simulink library "modularPlant_cl"  (R2018b)
settings: Solver=VariableStepAuto  StartTime=0.0  StopTime=10.0  RelTol=1e-3
libraries: groundStation_cl x1, tethers_cl x1, vehicle_cl x1, winch_cl x1
settings Model: Creator=mcobb  LastModifiedBy=mcobb

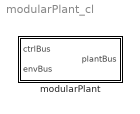
== system modularPlant_cl ==
  modularPlant : Subsystem  VariantControl=VSS_plant_modularPlant

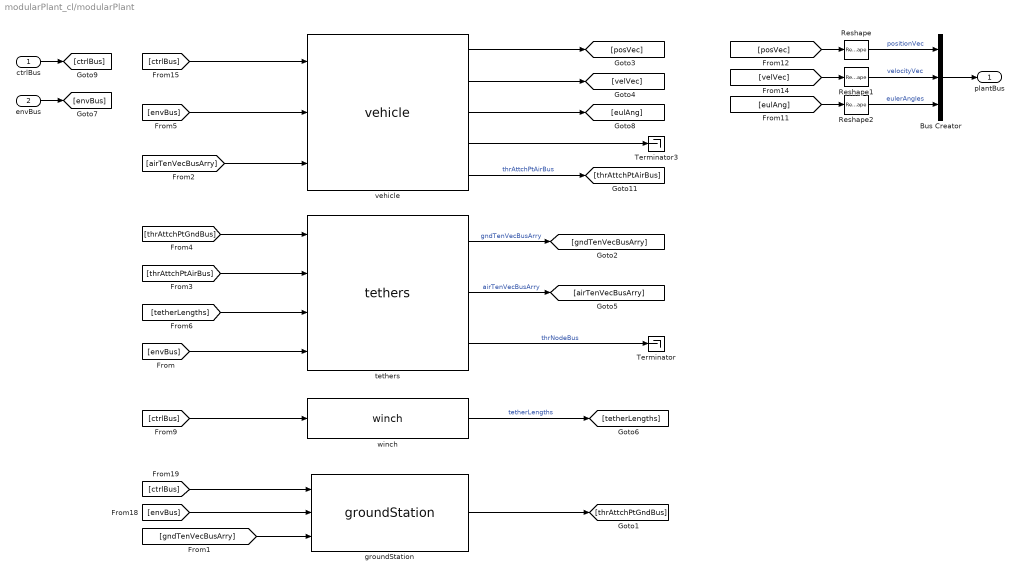
== system modularPlant_cl/modularPlant ==
  ctrlBus : Inport  OutDataTypeStr=Bus: ctrlBus
  envBus : Inport  Port=2  OutDataTypeStr=Bus: envBus
  Bus Creator : BusCreator  Inputs=3  OutDataTypeStr=Bus: plantBus
  Reshape : Reshape  OutputDimensionality=Column vector (2-D)
  Reshape1 : Reshape  OutputDimensionality=Column vector (2-D)
  Reshape2 : Reshape  OutputDimensionality=Column vector (2-D)
  Terminator : Terminator
  Terminator3 : Terminator
  groundStation : groundStation_cl/groundStation  SystemSampleTime=-1
  "tethers " : tethers_cl/tethers  SystemSampleTime=-1
  vehicle : vehicle_cl/vehicle  SystemSampleTime=-1
  winch : winch_cl/winch  SystemSampleTime=-1
  plantBus : Outport  OutDataTypeStr=Bus: plantBus
  wires:
  envBus/1 -> [envBus]
  ctrlBus/1 -> [ctrlBus]
  Bus Creator/1 -> plantBus/1
  Reshape/1 -> Bus Creator/1  "positionVec"
  Reshape2/1 -> Bus Creator/3  "eulerAngles"
  Reshape1/1 -> Bus Creator/2  "velocityVec"
  winch/1 -> [tetherLengths]  "tetherLengths"
  [posVec] -> Reshape/1
  [velVec] -> Reshape1/1
  [eulAng] -> Reshape2/1
  vehicle/3 -> [eulAng]
  vehicle/1 -> [posVec]
  vehicle/5 -> [thrAttchPtAirBus]  "thrAttchPtAirBus"
  vehicle/2 -> [velVec]
  vehicle/4 -> Terminator3/1
  [envBus] -> "tethers "/4
  groundStation/1 -> [thrAttchPtGndBus]
  "tethers "/1 -> [gndTenVecBusArry]  "gndTenVecBusArry"
  "tethers "/2 -> [airTenVecBusArry]  "airTenVecBusArry"
  "tethers "/3 -> Terminator/1  "thrNodeBus"
  [gndTenVecBusArry] -> groundStation/3
  [airTenVecBusArry] -> vehicle/3
  [thrAttchPtAirBus] -> "tethers "/2
  [thrAttchPtGndBus] -> "tethers "/1
  [tetherLengths] -> "tethers "/3
  [envBus] -> groundStation/2
  [ctrlBus] -> groundStation/1
  [ctrlBus] -> vehicle/1
  [envBus] -> vehicle/2
  [ctrlBus] -> winch/1
